simulink model "fengnengmoxing"  (R2014a)
settings: Solver=ode45  StartTime=0.0  StopTime=5000  RelTol=1e-3
libraries: simulink x1
settings Model: Creator=hsinwang  LastModifiedBy=hsinwang

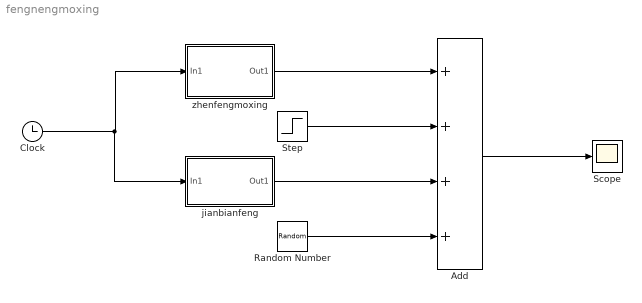
== system fengnengmoxing ==
  Add : Sum  Inputs=++++
  Clock : Clock
  Random Number : RandomNumber  SampleTime=0.1
  Scope : Scope
      settings: YMin=9  YMax=19
  Step : Step  SampleTime=0
  jianbianfeng : Subsystem
  "zhenfengmoxing " : Subsystem
  wires:
  Clock/1 -> jianbianfeng/1(In1), "zhenfengmoxing "/1(In1)
  "zhenfengmoxing "/1(Out1) -> Add/1
  Step/1 -> Add/2
  Add/1 -> Scope/1
  Random Number/1 -> Add/4
  jianbianfeng/1(Out1) -> Add/3

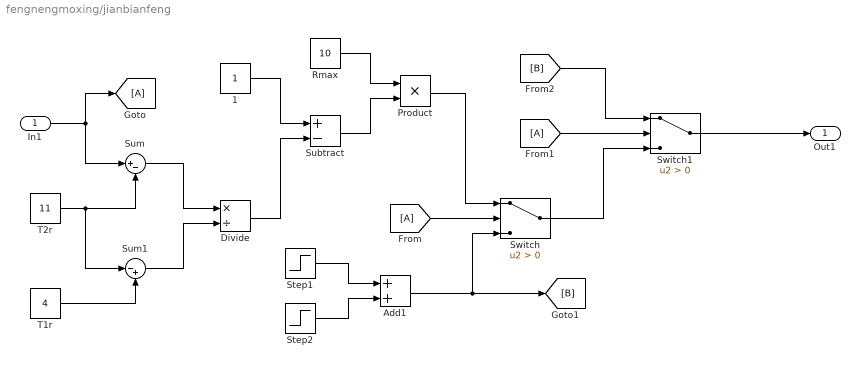
== system fengnengmoxing/jianbianfeng ==
  In1 : Inport
  1 : Constant
  Add1 : Sum
  Divide : Product  Inputs=*/
  Product : Product
  "Rmax " : Constant  Value=10
  Step1 : Step  SampleTime=0
  Step2 : Step  SampleTime=0
  Subtract : Sum  Inputs=+-
  Sum : Sum  Inputs=|+-
  Sum1 : Sum  Inputs=|-+
  Switch : Switch  Criteria=u2 > Threshold
  Switch1 : Switch  Criteria=u2 > Threshold
  "T1r " : Constant  Value=4
  "T2r " : Constant  Value=11
  Out1 : Outport
  wires:
  Step2/1 -> Add1/2
  Step1/1 -> Add1/1
  [A] -> Switch1/2
  1/1 -> Subtract/1
  Product/1 -> Switch/1
  Sum/1 -> Divide/1
  Switch1/1 -> Out1/1
  Divide/1 -> Subtract/2
  Add1/1 -> Switch/3, [B]
  Sum1/1 -> Divide/2
  [B] -> Switch1/1
  [A] -> Switch/2
  "T1r "/1 -> Sum1/2
  "Rmax "/1 -> Product/1
  "T2r "/1 -> Sum1/1, Sum/2
  Subtract/1 -> Product/2
  Switch/1 -> Switch1/3
  In1/1 -> Sum/1, [A]

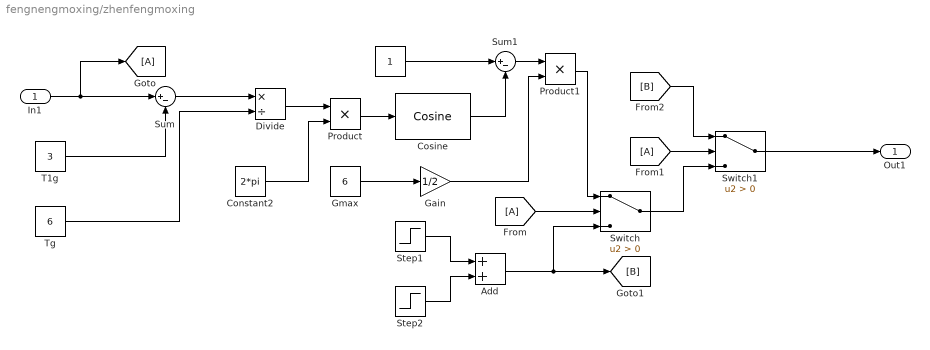
== system fengnengmoxing/zhenfengmoxing  ==
  In1 : Inport
  " Gmax " : Constant  Value=6
  " " : Constant
  Add : Sum
  Constant2 : Constant  Value=2*pi
  Cosine : simulink/Lookup Tables/Cosine  Formula=cos(2*pi*u)  NumDataPoints=(2^5)+1  OutputWordLength=16  InternalRulePriority=Speed
  Divide : Product  Inputs=*/
  Gain : Gain  Gain=1/2
  Product : Product
  Product1 : Product
  Step1 : Step  SampleTime=0
  Step2 : Step  SampleTime=0
  Sum : Sum  Inputs=|+-
  Sum1 : Sum  Inputs=|+-
  Switch : Switch  Criteria=u2 > Threshold
  Switch1 : Switch  Criteria=u2 > Threshold
  "T1g " : Constant  Value=3
  "Tg " : Constant  Value=6
  Out1 : Outport
  wires:
  Product/1 -> Cosine/1
  Divide/1 -> Product/1
  Constant2/1 -> Product/2
  Sum/1 -> Divide/1
  "T1g "/1 -> Sum/2
  In1/1 -> Sum/1, [A]
  "Tg "/1 -> Divide/2
  Cosine/1 -> Sum1/2
  Product1/1 -> Switch/1
  Sum1/1 -> Product1/1
  Gain/1 -> Product1/2
  Switch/1 -> Switch1/3
  " Gmax "/1 -> Gain/1
  Step1/1 -> Add/1
  " "/1 -> Sum1/1
  Step2/1 -> Add/2
  Switch1/1 -> Out1/1
  Add/1 -> [B], Switch/3
  [A] -> Switch/2
  [A] -> Switch1/2
  [B] -> Switch1/1
